simulink model "IEEE14_case"  (R2024b)
settings: Solver=FixedStepAuto  StartTime=0  StopTime=2  FixedStep=1e-7  RelTol=1e-3
values from neighbouring files (symbols this model uses):
  GFL_15_Bva = 0.009    [IEEE14_parameters.m]
  GFL_15_C_bus_pu = 7.179419    [IEEE14_parameters.m]
  GFL_15_f0 = 60    [IEEE14_parameters.m]
  GFL_15_I_id = 691.26967    [IEEE14_parameters.m]
  GFL_15_I_iq = 691.26967    [IEEE14_parameters.m]
  GFL_15_I_od = 45.2207    [IEEE14_parameters.m]
  GFL_15_I_oq = 45.2207    [IEEE14_parameters.m]
  GFL_15_I_pll = 0.78    [IEEE14_parameters.m]
  GFL_15_Kdi = 0.09    [IEEE14_parameters.m]
  GFL_15_Kdo = 0.9    [IEEE14_parameters.m]
  GFL_15_Kqi = 0.09    [IEEE14_parameters.m]
  GFL_15_Kqo = 0.9    [IEEE14_parameters.m]
  GFL_15_Lg_pu = 0.631447    [IEEE14_parameters.m]
  GFL_15_mode = 1    [IEEE14_parameters.m]
  GFL_15_P_id = 3.7166    [IEEE14_parameters.m]
  GFL_15_P_iq = 3.7166    [IEEE14_parameters.m]
  GFL_15_P_od = 0.4798    [IEEE14_parameters.m]
  GFL_15_P_oq = 0.4798    [IEEE14_parameters.m]
  GFL_15_P_pll = 290.42    [IEEE14_parameters.m]
  GFL_15_Qe_ref = 0.2    [IEEE14_parameters.m]
  GFL_15_Rg_pu = 0.024016    [IEEE14_parameters.m]
  GFL_15_Sbase = 1.000000e+4    (= 10000)    [IEEE14_parameters.m]
  GFL_15_Tdi = 0.01    [IEEE14_parameters.m]
  GFL_15_Tdo = 0.2    [IEEE14_parameters.m]
  GFL_15_Tqi = 0.01    [IEEE14_parameters.m]
  GFL_15_Tqo = 0.2    [IEEE14_parameters.m]
  GFL_15_Vbase = 380    [IEEE14_parameters.m]
  GFL_15_Vdc_ref = 1.011475    [IEEE14_parameters.m]
  GFL_15_Vdcbase = 700    [IEEE14_parameters.m]
  GFL_15_vq_ref = 0    [IEEE14_parameters.m]
  GFL_16_Bva = 0.002    [IEEE14_parameters.m]
  GFL_16_C_bus_pu = 7.179419    [IEEE14_parameters.m]
  GFL_16_f0 = 60    [IEEE14_parameters.m]
  GFL_16_I_id = 691.26967    [IEEE14_parameters.m]
  GFL_16_I_iq = 691.26967    [IEEE14_parameters.m]
  GFL_16_I_od = 45.2207    [IEEE14_parameters.m]
  GFL_16_I_oq = 45.2207    [IEEE14_parameters.m]
  GFL_16_I_pll = 0.78    [IEEE14_parameters.m]
  GFL_16_Kdi = 0.05    [IEEE14_parameters.m]
  GFL_16_Kdo = 0.5    [IEEE14_parameters.m]
  GFL_16_Kqi = 0.05    [IEEE14_parameters.m]
  GFL_16_Kqo = 0.5    [IEEE14_parameters.m]
  GFL_16_Lg_pu = 0.631447    [IEEE14_parameters.m]
  GFL_16_mode = 1    [IEEE14_parameters.m]
  GFL_16_P_id = 3.7166    [IEEE14_parameters.m]
  GFL_16_P_iq = 3.7166    [IEEE14_parameters.m]
  GFL_16_P_od = 0.4798    [IEEE14_parameters.m]
  GFL_16_P_oq = 0.4798    [IEEE14_parameters.m]
  GFL_16_P_pll = 290.42    [IEEE14_parameters.m]
  GFL_16_Qe_ref = 0.2    [IEEE14_parameters.m]
  GFL_16_Rg_pu = 0.024016    [IEEE14_parameters.m]
  GFL_16_Sbase = 1.000000e+4    (= 10000)    [IEEE14_parameters.m]
  GFL_16_Tdi = 0.01    [IEEE14_parameters.m]
  GFL_16_Tdo = 0.2    [IEEE14_parameters.m]
  GFL_16_Tqi = 0.01    [IEEE14_parameters.m]
  GFL_16_Tqo = 0.2    [IEEE14_parameters.m]
  GFL_16_Vbase = 380    [IEEE14_parameters.m]
  GFL_16_Vdc_ref = 1.01144    [IEEE14_parameters.m]
  GFL_16_Vdcbase = 700    [IEEE14_parameters.m]
  GFL_16_vq_ref = 0    [IEEE14_parameters.m]
  GFL_17_Bva = 0.002    [IEEE14_parameters.m]
  GFL_17_C_bus_pu = 7.179419    [IEEE14_parameters.m]
  GFL_17_f0 = 60    [IEEE14_parameters.m]
  GFL_17_I_id = 691.26967    [IEEE14_parameters.m]
  GFL_17_I_iq = 691.26967    [IEEE14_parameters.m]
  GFL_17_I_od = 45.2207    [IEEE14_parameters.m]
  GFL_17_I_oq = 45.2207    [IEEE14_parameters.m]
  GFL_17_I_pll = 0.78    [IEEE14_parameters.m]
  GFL_17_Kdi = 0.05    [IEEE14_parameters.m]
  GFL_17_Kdo = 0.5    [IEEE14_parameters.m]
  GFL_17_Kqi = 0.05    [IEEE14_parameters.m]
  GFL_17_Kqo = 0.5    [IEEE14_parameters.m]
  GFL_17_Lg_pu = 0.631447    [IEEE14_parameters.m]
  GFL_17_mode = 1    [IEEE14_parameters.m]
  GFL_17_P_id = 3.7166    [IEEE14_parameters.m]
  GFL_17_P_iq = 3.7166    [IEEE14_parameters.m]
  GFL_17_P_od = 0.4798    [IEEE14_parameters.m]
  GFL_17_P_oq = 0.4798    [IEEE14_parameters.m]
  GFL_17_P_pll = 290.42    [IEEE14_parameters.m]
  GFL_17_Qe_ref = 0.2    [IEEE14_parameters.m]
  GFL_17_Rg_pu = 0.024016    [IEEE14_parameters.m]
  GFL_17_Sbase = 1.000000e+4    (= 10000)    [IEEE14_parameters.m]
  GFL_17_Tdi = 0.01    [IEEE14_parameters.m]
  GFL_17_Tdo = 0.2    [IEEE14_parameters.m]
  GFL_17_Tqi = 0.01    [IEEE14_parameters.m]
  GFL_17_Tqo = 0.2    [IEEE14_parameters.m]
  GFL_17_Vbase = 380    [IEEE14_parameters.m]
  GFL_17_Vdc_ref = 1.011632    [IEEE14_parameters.m]
  GFL_17_Vdcbase = 700    [IEEE14_parameters.m]
  GFL_17_vq_ref = 0    [IEEE14_parameters.m]
  GFL_18_Bva = 0.002    [IEEE14_parameters.m]
  GFL_18_C_bus_pu = 7.179419    [IEEE14_parameters.m]
  GFL_18_f0 = 60    [IEEE14_parameters.m]
  GFL_18_I_id = 691.26967    [IEEE14_parameters.m]
  GFL_18_I_iq = 691.26967    [IEEE14_parameters.m]
  GFL_18_I_od = 45.2207    [IEEE14_parameters.m]
  GFL_18_I_oq = 45.2207    [IEEE14_parameters.m]
  GFL_18_I_pll = 0.78    [IEEE14_parameters.m]
  GFL_18_Kdi = 0.05    [IEEE14_parameters.m]
  GFL_18_Kdo = 0.5    [IEEE14_parameters.m]
  GFL_18_Kqi = 0.05    [IEEE14_parameters.m]
  GFL_18_Kqo = 0.5    [IEEE14_parameters.m]
  GFL_18_Lg_pu = 0.631447    [IEEE14_parameters.m]
  GFL_18_mode = 1    [IEEE14_parameters.m]
  GFL_18_P_id = 3.7166    [IEEE14_parameters.m]
  GFL_18_P_iq = 3.7166    [IEEE14_parameters.m]
  GFL_18_P_od = 0.4798    [IEEE14_parameters.m]
  GFL_18_P_oq = 0.4798    [IEEE14_parameters.m]
  GFL_18_P_pll = 290.42    [IEEE14_parameters.m]
  GFL_18_Qe_ref = 0.2    [IEEE14_parameters.m]
  GFL_18_Rg_pu = 0.024016    [IEEE14_parameters.m]
  GFL_18_Sbase = 1.000000e+4    (= 10000)    [IEEE14_parameters.m]
  GFL_18_Tdi = 0.01    [IEEE14_parameters.m]
  GFL_18_Tdo = 0.2    [IEEE14_parameters.m]
  GFL_18_Tqi = 0.01    [IEEE14_parameters.m]
  GFL_18_Tqo = 0.2    [IEEE14_parameters.m]
  GFL_18_Vbase = 380    [IEEE14_parameters.m]
  GFL_18_Vdc_ref = 1.011572    [IEEE14_parameters.m]
  GFL_18_Vdcbase = 700    [IEEE14_parameters.m]
  GFL_18_vq_ref = 0    [IEEE14_parameters.m]
  ... (+180 more)
(part 4 of 25)

== system IEEE14_case/SG_D_1 ==
  v_d_SG_D_1 : Inport
  v_q_SG_D_1 : Inport  Port=2
  E_fd_SG_D_1 : Integrator  InitialCondition=3.4212573415419114
  Px_1_SG_D_1 : Integrator  InitialCondition=0.0
  Px_2_SG_D_1 : Integrator  InitialCondition=0.0
  Px_3_SG_D_1 : Integrator  InitialCondition=-3.1830279294144415e-26
  R_f_SG_D_1 : Integrator  InitialCondition=23.098374565895817
  T_e_SG_D_1_block : Subsystem
  T_m_SG_D_1 : Integrator  InitialCondition=1.9014466706454893
  V_f_SG_D_1 : Integrator  InitialCondition=34.212573415419115
  d_E_fd_SG_D_1_block : Subsystem
  d_Px_1_SG_D_1_block : Subsystem
  d_Px_2_SG_D_1_block : Subsystem
  d_Px_3_SG_D_1_block : Subsystem
  d_R_f_SG_D_1_block : Subsystem
  d_T_m_SG_D_1_block : Subsystem
  d_V_f_SG_D_1_block : Subsystem
  d_psi_1d_SG_D_1_block : Subsystem
  d_psi_d_SG_D_1_block : Subsystem
  d_psi_fd_SG_D_1_block : Subsystem
  d_psi_gq_SG_D_1_block : Subsystem
  d_psi_kq_SG_D_1_block : Subsystem
  d_psi_q_SG_D_1_block : Subsystem
  d_theta_SG_D_1_block : Subsystem
  d_w_SG_D_1_block : Subsystem
  i_d_SG_D_1_block : Subsystem
  i_q_SG_D_1_block : Subsystem
  psi_1d_SG_D_1 : Integrator  InitialCondition=0.4032623891736521
  psi_d_SG_D_1 : Integrator  InitialCondition=0.32169495802856396
  psi_fd_SG_D_1 : Integrator  InitialCondition=0.8143622421448962
  psi_gq_SG_D_1 : Integrator  InitialCondition=0.6228002528652177
  psi_kq_SG_D_1 : Integrator  InitialCondition=-0.9731253951019027
  psi_q_SG_D_1 : Integrator  InitialCondition=-1.0120504109059787
  theta_SG_D_1 : Integrator  InitialCondition=1.263285946581872
  theta_SG_D_1_out_block : Subsystem
  w_SG_D_1 : Integrator  InitialCondition=376.99111843077515
  w_SG_D_1_out_block : Subsystem
  i_d_SG_D_1 : Outport
  i_q_SG_D_1 : Outport  Port=2
  T_e_SG_D_1 : Outport  Port=3
  w_SG_D_1_out : Outport  Port=4
  theta_SG_D_1_out : Outport  Port=5
  wires:
  d_theta_SG_D_1_block/1(Blockout_d_theta_SG_D_1_10b81) -> theta_SG_D_1/1
  V_f_SG_D_1/1 -> d_V_f_SG_D_1_block/14(State_V_f_SG_D_1_9a6da), d_E_fd_SG_D_1_block/2(State_V_f_SG_D_1_aa35b)
  psi_kq_SG_D_1/1 -> d_psi_q_SG_D_1_block/2(State_psi_kq_SG_D_1_494df), d_psi_gq_SG_D_1_block/3(State_psi_kq_SG_D_1_80cf5), d_psi_kq_SG_D_1_block/4(State_psi_kq_SG_D_1_7d6ac), d_psi_gq_SG_D_1_block/5(State_psi_kq_SG_D_1_884a1), d_V_f_SG_D_1_block/10(State_psi_kq_SG_D_1_02ae0), d_psi_gq_SG_D_1_block/8(State_psi_kq_SG_D_1_12411), i_d_SG_D_1_block/2(State_psi_kq_SG_D_1_0b4c3), d_psi_kq_SG_D_1_block/2(State_psi_kq_SG_D_1_b5070), T_e_SG_D_1_block/3(State_psi_kq_SG_D_1_246e1), i_q_SG_D_1_block/2(State_psi_kq_SG_D_1_fbc68), d_w_SG_D_1_block/5(State_psi_kq_SG_D_1_9c615)
  w_SG_D_1_out_block/1(Blockout_w_SG_D_1_out_d4c3b) -> w_SG_D_1_out/1
  d_Px_1_SG_D_1_block/1(Blockout_d_Px_1_SG_D_1_a4a61) -> Px_1_SG_D_1/1
  w_SG_D_1/1 -> d_V_f_SG_D_1_block/8(State_w_SG_D_1_7c0e0), d_psi_q_SG_D_1_block/9(State_w_SG_D_1_856b5), d_psi_d_SG_D_1_block/9(State_w_SG_D_1_7866a), d_V_f_SG_D_1_block/13(State_w_SG_D_1_d278a), d_T_m_SG_D_1_block/1(State_w_SG_D_1_4fd49), d_theta_SG_D_1_block/1(State_w_SG_D_1_d1dcd), d_Px_1_SG_D_1_block/2(State_w_SG_D_1_183d0), d_Px_2_SG_D_1_block/4(State_w_SG_D_1_83c31), d_w_SG_D_1_block/1(State_w_SG_D_1_bf0fb), d_Px_3_SG_D_1_block/6(State_w_SG_D_1_d6c43), w_SG_D_1_out_block/1(State_w_SG_D_1_b42d2)
  d_T_m_SG_D_1_block/1(Blockout_d_T_m_SG_D_1_8a3f6) -> T_m_SG_D_1/1
  d_Px_2_SG_D_1_block/1(Blockout_d_Px_2_SG_D_1_c2665) -> Px_2_SG_D_1/1
  d_Px_3_SG_D_1_block/1(Blockout_d_Px_3_SG_D_1_27eea) -> Px_3_SG_D_1/1
  psi_q_SG_D_1/1 -> d_psi_d_SG_D_1_block/8(State_psi_q_SG_D_1_339cd), d_psi_q_SG_D_1_block/3(State_psi_q_SG_D_1_68044), d_psi_gq_SG_D_1_block/6(State_psi_q_SG_D_1_99c8d), d_w_SG_D_1_block/7(State_psi_q_SG_D_1_36eb9), d_V_f_SG_D_1_block/11(State_psi_q_SG_D_1_7b289), i_d_SG_D_1_block/3(State_psi_q_SG_D_1_e8ece), d_w_SG_D_1_block/6(State_psi_q_SG_D_1_06dea), d_psi_gq_SG_D_1_block/9(State_psi_q_SG_D_1_31f88), i_q_SG_D_1_block/3(State_psi_q_SG_D_1_42b5e), d_V_f_SG_D_1_block/7(State_psi_q_SG_D_1_b21ce), d_psi_kq_SG_D_1_block/5(State_psi_q_SG_D_1_c6187), T_e_SG_D_1_block/4(State_psi_q_SG_D_1_fd30f), T_e_SG_D_1_block/5(State_psi_q_SG_D_1_04e42)
  psi_fd_SG_D_1/1 -> d_psi_fd_SG_D_1_block/2(State_psi_fd_SG_D_1_8f7d3), d_psi_fd_SG_D_1_block/10(State_psi_fd_SG_D_1_86724), d_psi_fd_SG_D_1_block/4(State_psi_fd_SG_D_1_d976b), d_psi_fd_SG_D_1_block/7(State_psi_fd_SG_D_1_c7a2f), d_psi_d_SG_D_1_block/3(State_psi_fd_SG_D_1_aad83), d_psi_1d_SG_D_1_block/5(State_psi_fd_SG_D_1_15435), d_w_SG_D_1_block/10(State_psi_fd_SG_D_1_a5e83), i_d_SG_D_1_block/7(State_psi_fd_SG_D_1_51096), i_q_SG_D_1_block/7(State_psi_fd_SG_D_1_ad572), d_V_f_SG_D_1_block/6(State_psi_fd_SG_D_1_fca9a), T_e_SG_D_1_block/8(State_psi_fd_SG_D_1_a5ec6), d_psi_1d_SG_D_1_block/2(State_psi_fd_SG_D_1_00af5)
  psi_gq_SG_D_1/1 -> d_psi_q_SG_D_1_block/1(State_psi_gq_SG_D_1_af930), d_psi_gq_SG_D_1_block/1(State_psi_gq_SG_D_1_6811c), d_psi_gq_SG_D_1_block/2(State_psi_gq_SG_D_1_53a5f), d_psi_gq_SG_D_1_block/7(State_psi_gq_SG_D_1_8041e), d_w_SG_D_1_block/4(State_psi_gq_SG_D_1_d212a), d_psi_kq_SG_D_1_block/1(State_psi_gq_SG_D_1_dba3b), i_d_SG_D_1_block/1(State_psi_gq_SG_D_1_8ae81), d_V_f_SG_D_1_block/9(State_psi_gq_SG_D_1_33342), d_psi_gq_SG_D_1_block/4(State_psi_gq_SG_D_1_5ed70), T_e_SG_D_1_block/2(State_psi_gq_SG_D_1_b91dd), i_q_SG_D_1_block/1(State_psi_gq_SG_D_1_70f72), d_psi_kq_SG_D_1_block/3(State_psi_gq_SG_D_1_cd69f)
  v_d_SG_D_1/1 -> d_psi_d_SG_D_1_block/4(Input_v_d_SG_D_1_751e0), d_psi_q_SG_D_1_block/4(Input_v_d_SG_D_1_3462f)
  T_m_SG_D_1/1 -> d_T_m_SG_D_1_block/2(State_T_m_SG_D_1_4e3cf), d_w_SG_D_1_block/2(State_T_m_SG_D_1_e0642)
  v_q_SG_D_1/1 -> d_psi_d_SG_D_1_block/6(Input_v_q_SG_D_1_569c6), d_psi_q_SG_D_1_block/6(Input_v_q_SG_D_1_86d27)
  Px_1_SG_D_1/1 -> d_Px_1_SG_D_1_block/1(State_Px_1_SG_D_1_41b99), d_Px_2_SG_D_1_block/3(State_Px_1_SG_D_1_ca7d0), d_Px_3_SG_D_1_block/4(State_Px_1_SG_D_1_d599f), d_Px_3_SG_D_1_block/5(State_Px_1_SG_D_1_5257c), d_Px_2_SG_D_1_block/2(State_Px_1_SG_D_1_02194)
  theta_SG_D_1/1 -> d_psi_d_SG_D_1_block/5(State_theta_SG_D_1_5b2d6), d_psi_q_SG_D_1_block/7(State_theta_SG_D_1_4261b), i_d_SG_D_1_block/4(State_theta_SG_D_1_02ca1), d_psi_d_SG_D_1_block/7(State_theta_SG_D_1_7d7a3), i_q_SG_D_1_block/4(State_theta_SG_D_1_4335e), d_psi_q_SG_D_1_block/5(State_theta_SG_D_1_16401), theta_SG_D_1_out_block/1(State_theta_SG_D_1_c8a88), i_q_SG_D_1_block/8(State_theta_SG_D_1_fd587), i_d_SG_D_1_block/8(State_theta_SG_D_1_8959d)
  Px_2_SG_D_1/1 -> d_Px_2_SG_D_1_block/1(State_Px_2_SG_D_1_52166), d_Px_3_SG_D_1_block/2(State_Px_2_SG_D_1_173b9), d_Px_3_SG_D_1_block/3(State_Px_2_SG_D_1_5b4c4)
  psi_d_SG_D_1/1 -> d_psi_fd_SG_D_1_block/9(State_psi_d_SG_D_1_5418d), d_psi_d_SG_D_1_block/2(State_psi_d_SG_D_1_b0cbd), d_psi_q_SG_D_1_block/8(State_psi_d_SG_D_1_ad817), d_w_SG_D_1_block/9(State_psi_d_SG_D_1_eab0d), d_w_SG_D_1_block/3(State_psi_d_SG_D_1_3bbbe), d_V_f_SG_D_1_block/5(State_psi_d_SG_D_1_3c550), d_psi_1d_SG_D_1_block/4(State_psi_d_SG_D_1_719b4), i_d_SG_D_1_block/6(State_psi_d_SG_D_1_e218a), i_q_SG_D_1_block/6(State_psi_d_SG_D_1_986bb), T_e_SG_D_1_block/1(State_psi_d_SG_D_1_5a569), d_V_f_SG_D_1_block/12(State_psi_d_SG_D_1_3754c), d_psi_fd_SG_D_1_block/6(State_psi_d_SG_D_1_eef22), T_e_SG_D_1_block/7(State_psi_d_SG_D_1_dfbb8)
  d_E_fd_SG_D_1_block/1(Blockout_d_E_fd_SG_D_1_7b54f) -> E_fd_SG_D_1/1
  psi_1d_SG_D_1/1 -> d_psi_fd_SG_D_1_block/3(State_psi_1d_SG_D_1_1898e), d_psi_fd_SG_D_1_block/8(State_psi_1d_SG_D_1_2c9f9), d_psi_d_SG_D_1_block/1(State_psi_1d_SG_D_1_69d00), d_psi_1d_SG_D_1_block/3(State_psi_1d_SG_D_1_c5f75), d_V_f_SG_D_1_block/4(State_psi_1d_SG_D_1_6838f), i_d_SG_D_1_block/5(State_psi_1d_SG_D_1_6fa9d), d_w_SG_D_1_block/8(State_psi_1d_SG_D_1_bb43d), i_q_SG_D_1_block/5(State_psi_1d_SG_D_1_63ddd), d_psi_1d_SG_D_1_block/1(State_psi_1d_SG_D_1_959f0), T_e_SG_D_1_block/6(State_psi_1d_SG_D_1_ba9b8), d_psi_fd_SG_D_1_block/5(State_psi_1d_SG_D_1_f6ad7)
  d_V_f_SG_D_1_block/1(Blockout_d_V_f_SG_D_1_61597) -> V_f_SG_D_1/1
  d_psi_q_SG_D_1_block/1(Blockout_d_psi_q_SG_D_1_f8953) -> psi_q_SG_D_1/1
  d_psi_gq_SG_D_1_block/1(Blockout_d_psi_gq_SG_D_1_56070) -> psi_gq_SG_D_1/1
  theta_SG_D_1_out_block/1(Blockout_theta_SG_D_1_out_3d7c0) -> theta_SG_D_1_out/1
  d_R_f_SG_D_1_block/1(Blockout_d_R_f_SG_D_1_dc367) -> R_f_SG_D_1/1
  d_w_SG_D_1_block/1(Blockout_d_w_SG_D_1_3fcfa) -> w_SG_D_1/1
  T_e_SG_D_1_block/1(Blockout_T_e_SG_D_1_52337) -> T_e_SG_D_1/1
  d_psi_d_SG_D_1_block/1(Blockout_d_psi_d_SG_D_1_2cdbf) -> psi_d_SG_D_1/1
  d_psi_kq_SG_D_1_block/1(Blockout_d_psi_kq_SG_D_1_d51b4) -> psi_kq_SG_D_1/1
  i_q_SG_D_1_block/1(Blockout_i_q_SG_D_1_04b1b) -> i_q_SG_D_1/1
  i_d_SG_D_1_block/1(Blockout_i_d_SG_D_1_f5e95) -> i_d_SG_D_1/1
  d_psi_1d_SG_D_1_block/1(Blockout_d_psi_1d_SG_D_1_ce82a) -> psi_1d_SG_D_1/1
  Px_3_SG_D_1/1 -> d_V_f_SG_D_1_block/3(State_Px_3_SG_D_1_35ab0), d_Px_3_SG_D_1_block/1(State_Px_3_SG_D_1_65e83)
  R_f_SG_D_1/1 -> d_V_f_SG_D_1_block/2(State_R_f_SG_D_1_39127), d_R_f_SG_D_1_block/2(State_R_f_SG_D_1_c9358)
  E_fd_SG_D_1/1 -> d_V_f_SG_D_1_block/1(State_E_fd_SG_D_1_b54d1), d_E_fd_SG_D_1_block/1(State_E_fd_SG_D_1_314b1), d_R_f_SG_D_1_block/1(State_E_fd_SG_D_1_43088), d_psi_fd_SG_D_1_block/1(State_E_fd_SG_D_1_05819)
  d_psi_fd_SG_D_1_block/1(Blockout_d_psi_fd_SG_D_1_936e9) -> psi_fd_SG_D_1/1

== system IEEE14_case/SG_D_2 ==
  v_d_SG_D_2 : Inport
  v_q_SG_D_2 : Inport  Port=2
  E_fd_SG_D_2 : Integrator  InitialCondition=1.1780887532081583
  Px_1_SG_D_2 : Integrator  InitialCondition=0.0
  Px_2_SG_D_2 : Integrator  InitialCondition=0.0
  Px_3_SG_D_2 : Integrator  InitialCondition=-1.1116920340485189e-30
  R_f_SG_D_2 : Integrator  InitialCondition=7.953782068088223
  T_e_SG_D_2_block : Subsystem
  T_m_SG_D_2 : Integrator  InitialCondition=0.40016203494093494
  V_f_SG_D_2 : Integrator  InitialCondition=11.780887532081582
  d_E_fd_SG_D_2_block : Subsystem
  d_Px_1_SG_D_2_block : Subsystem
  d_Px_2_SG_D_2_block : Subsystem
  d_Px_3_SG_D_2_block : Subsystem
  d_R_f_SG_D_2_block : Subsystem
  d_T_m_SG_D_2_block : Subsystem
  d_V_f_SG_D_2_block : Subsystem
  d_psi_1d_SG_D_2_block : Subsystem
  d_psi_d_SG_D_2_block : Subsystem
  d_psi_fd_SG_D_2_block : Subsystem
  d_psi_gq_SG_D_2_block : Subsystem
  d_psi_kq_SG_D_2_block : Subsystem
  d_psi_q_SG_D_2_block : Subsystem
  d_theta_SG_D_2_block : Subsystem
  d_w_SG_D_2_block : Subsystem
  i_d_SG_D_2_block : Subsystem
  i_q_SG_D_2_block : Subsystem
  psi_1d_SG_D_2 : Integrator  InitialCondition=0.9389092187130986
  psi_d_SG_D_2 : Integrator  InitialCondition=0.9324449069699886
  psi_fd_SG_D_2 : Integrator  InitialCondition=0.9714893498983717
  psi_gq_SG_D_2 : Integrator  InitialCondition=0.290890212850531
  psi_kq_SG_D_2 : Integrator  InitialCondition=-0.45451595757895474
  psi_q_SG_D_2 : Integrator  InitialCondition=-0.47269659588211294
  theta_SG_D_2 : Integrator  InitialCondition=0.39900394090305374
  theta_SG_D_2_out_block : Subsystem
  w_SG_D_2 : Integrator  InitialCondition=376.99111843077515
  w_SG_D_2_out_block : Subsystem
  i_d_SG_D_2 : Outport
  i_q_SG_D_2 : Outport  Port=2
  T_e_SG_D_2 : Outport  Port=3
  w_SG_D_2_out : Outport  Port=4
  theta_SG_D_2_out : Outport  Port=5
  wires:
  T_e_SG_D_2_block/1(Blockout_T_e_SG_D_2_7a393) -> T_e_SG_D_2/1
  d_Px_2_SG_D_2_block/1(Blockout_d_Px_2_SG_D_2_dd680) -> Px_2_SG_D_2/1
  d_T_m_SG_D_2_block/1(Blockout_d_T_m_SG_D_2_a859c) -> T_m_SG_D_2/1
  w_SG_D_2/1 -> d_psi_d_SG_D_2_block/9(State_w_SG_D_2_3bf29), d_w_SG_D_2_block/1(State_w_SG_D_2_04eee), d_V_f_SG_D_2_block/8(State_w_SG_D_2_66c76), d_psi_q_SG_D_2_block/9(State_w_SG_D_2_ecb88), d_V_f_SG_D_2_block/13(State_w_SG_D_2_ea751), d_theta_SG_D_2_block/1(State_w_SG_D_2_44e1a), d_T_m_SG_D_2_block/1(State_w_SG_D_2_28412), d_Px_2_SG_D_2_block/4(State_w_SG_D_2_0c27f), d_Px_3_SG_D_2_block/6(State_w_SG_D_2_29f15), d_Px_1_SG_D_2_block/2(State_w_SG_D_2_57c67), w_SG_D_2_out_block/1(State_w_SG_D_2_35bfa)
  psi_q_SG_D_2/1 -> d_psi_d_SG_D_2_block/8(State_psi_q_SG_D_2_54a7c), d_psi_q_SG_D_2_block/3(State_psi_q_SG_D_2_b05c7), d_psi_gq_SG_D_2_block/6(State_psi_q_SG_D_2_c887c), d_psi_gq_SG_D_2_block/9(State_psi_q_SG_D_2_400a1), d_psi_kq_SG_D_2_block/5(State_psi_q_SG_D_2_cfb7c), d_w_SG_D_2_block/7(State_psi_q_SG_D_2_8635e), d_V_f_SG_D_2_block/7(State_psi_q_SG_D_2_698d7), i_d_SG_D_2_block/3(State_psi_q_SG_D_2_b30b5), T_e_SG_D_2_block/4(State_psi_q_SG_D_2_7be04), i_q_SG_D_2_block/3(State_psi_q_SG_D_2_38e4d), d_w_SG_D_2_block/6(State_psi_q_SG_D_2_03373), T_e_SG_D_2_block/5(State_psi_q_SG_D_2_caf2c), d_V_f_SG_D_2_block/11(State_psi_q_SG_D_2_de371)
  w_SG_D_2_out_block/1(Blockout_w_SG_D_2_out_7dd39) -> w_SG_D_2_out/1
  T_m_SG_D_2/1 -> d_T_m_SG_D_2_block/2(State_T_m_SG_D_2_839d4), d_w_SG_D_2_block/2(State_T_m_SG_D_2_0748f)
  d_theta_SG_D_2_block/1(Blockout_d_theta_SG_D_2_e87fa) -> theta_SG_D_2/1
  d_Px_1_SG_D_2_block/1(Blockout_d_Px_1_SG_D_2_466a7) -> Px_1_SG_D_2/1
  d_Px_3_SG_D_2_block/1(Blockout_d_Px_3_SG_D_2_c9fb9) -> Px_3_SG_D_2/1
  Px_2_SG_D_2/1 -> d_Px_2_SG_D_2_block/1(State_Px_2_SG_D_2_863da), d_Px_3_SG_D_2_block/2(State_Px_2_SG_D_2_b3dc6), d_Px_3_SG_D_2_block/3(State_Px_2_SG_D_2_577d6)
  theta_SG_D_2/1 -> d_psi_d_SG_D_2_block/5(State_theta_SG_D_2_fba08), d_psi_q_SG_D_2_block/5(State_theta_SG_D_2_ba654), i_d_SG_D_2_block/4(State_theta_SG_D_2_acd34), d_psi_q_SG_D_2_block/7(State_theta_SG_D_2_5db71), i_d_SG_D_2_block/8(State_theta_SG_D_2_fc4e1), i_q_SG_D_2_block/4(State_theta_SG_D_2_4758d), i_q_SG_D_2_block/8(State_theta_SG_D_2_47d8a), theta_SG_D_2_out_block/1(State_theta_SG_D_2_36941), d_psi_d_SG_D_2_block/7(State_theta_SG_D_2_1738b)
  i_d_SG_D_2_block/1(Blockout_i_d_SG_D_2_ab50a) -> i_d_SG_D_2/1
  psi_d_SG_D_2/1 -> d_psi_fd_SG_D_2_block/6(State_psi_d_SG_D_2_1798b), d_psi_fd_SG_D_2_block/9(State_psi_d_SG_D_2_c30ab), d_psi_q_SG_D_2_block/8(State_psi_d_SG_D_2_4f2c3), d_psi_1d_SG_D_2_block/4(State_psi_d_SG_D_2_f297a), d_w_SG_D_2_block/3(State_psi_d_SG_D_2_6ae82), d_w_SG_D_2_block/9(State_psi_d_SG_D_2_d3800), d_psi_d_SG_D_2_block/2(State_psi_d_SG_D_2_46d33), d_V_f_SG_D_2_block/12(State_psi_d_SG_D_2_35745), i_d_SG_D_2_block/6(State_psi_d_SG_D_2_21b88), i_q_SG_D_2_block/6(State_psi_d_SG_D_2_afab4), d_V_f_SG_D_2_block/5(State_psi_d_SG_D_2_fc0d8), T_e_SG_D_2_block/1(State_psi_d_SG_D_2_5317f), T_e_SG_D_2_block/7(State_psi_d_SG_D_2_ed23a)
  psi_1d_SG_D_2/1 -> d_psi_fd_SG_D_2_block/5(State_psi_1d_SG_D_2_c8d78), d_psi_fd_SG_D_2_block/8(State_psi_1d_SG_D_2_e893c), d_psi_fd_SG_D_2_block/3(State_psi_1d_SG_D_2_84bab), d_psi_1d_SG_D_2_block/1(State_psi_1d_SG_D_2_5768c), d_V_f_SG_D_2_block/4(State_psi_1d_SG_D_2_cce5d), d_w_SG_D_2_block/8(State_psi_1d_SG_D_2_3458c), i_d_SG_D_2_block/5(State_psi_1d_SG_D_2_9c394), i_q_SG_D_2_block/5(State_psi_1d_SG_D_2_da86a), d_psi_d_SG_D_2_block/1(State_psi_1d_SG_D_2_d5455), T_e_SG_D_2_block/6(State_psi_1d_SG_D_2_2fd39), d_psi_1d_SG_D_2_block/3(State_psi_1d_SG_D_2_34f10)
  psi_kq_SG_D_2/1 -> d_psi_q_SG_D_2_block/2(State_psi_kq_SG_D_2_3a32d), d_psi_gq_SG_D_2_block/3(State_psi_kq_SG_D_2_229b6), d_psi_gq_SG_D_2_block/5(State_psi_kq_SG_D_2_a4801), d_psi_kq_SG_D_2_block/2(State_psi_kq_SG_D_2_f7bb1), d_V_f_SG_D_2_block/10(State_psi_kq_SG_D_2_9c81b), d_w_SG_D_2_block/5(State_psi_kq_SG_D_2_19d78), i_d_SG_D_2_block/2(State_psi_kq_SG_D_2_eeb5f), d_psi_kq_SG_D_2_block/4(State_psi_kq_SG_D_2_18fe7), i_q_SG_D_2_block/2(State_psi_kq_SG_D_2_485e8), d_psi_gq_SG_D_2_block/8(State_psi_kq_SG_D_2_c4824), T_e_SG_D_2_block/3(State_psi_kq_SG_D_2_8eee7)
  v_d_SG_D_2/1 -> d_psi_q_SG_D_2_block/4(Input_v_d_SG_D_2_1b10e), d_psi_d_SG_D_2_block/4(Input_v_d_SG_D_2_d6dc0)
  d_V_f_SG_D_2_block/1(Blockout_d_V_f_SG_D_2_c52b2) -> V_f_SG_D_2/1
  v_q_SG_D_2/1 -> d_psi_d_SG_D_2_block/6(Input_v_q_SG_D_2_00db2), d_psi_q_SG_D_2_block/6(Input_v_q_SG_D_2_876cf)
  Px_1_SG_D_2/1 -> d_Px_1_SG_D_2_block/1(State_Px_1_SG_D_2_416e3), d_Px_2_SG_D_2_block/2(State_Px_1_SG_D_2_cbeb2), d_Px_3_SG_D_2_block/4(State_Px_1_SG_D_2_b7377), d_Px_3_SG_D_2_block/5(State_Px_1_SG_D_2_616ef), d_Px_2_SG_D_2_block/3(State_Px_1_SG_D_2_01235)
  psi_fd_SG_D_2/1 -> d_psi_fd_SG_D_2_block/2(State_psi_fd_SG_D_2_2df35), d_psi_fd_SG_D_2_block/4(State_psi_fd_SG_D_2_f521e), d_psi_fd_SG_D_2_block/10(State_psi_fd_SG_D_2_fdcf2), d_psi_d_SG_D_2_block/3(State_psi_fd_SG_D_2_e734d), d_psi_fd_SG_D_2_block/7(State_psi_fd_SG_D_2_82c24), d_psi_1d_SG_D_2_block/5(State_psi_fd_SG_D_2_c105c), d_w_SG_D_2_block/10(State_psi_fd_SG_D_2_b728a), d_V_f_SG_D_2_block/6(State_psi_fd_SG_D_2_82b8b), i_d_SG_D_2_block/7(State_psi_fd_SG_D_2_34aa6), i_q_SG_D_2_block/7(State_psi_fd_SG_D_2_93752), d_psi_1d_SG_D_2_block/2(State_psi_fd_SG_D_2_4ee86), T_e_SG_D_2_block/8(State_psi_fd_SG_D_2_ca537)
  psi_gq_SG_D_2/1 -> d_psi_gq_SG_D_2_block/1(State_psi_gq_SG_D_2_f404a), d_psi_gq_SG_D_2_block/2(State_psi_gq_SG_D_2_79e41), d_psi_gq_SG_D_2_block/4(State_psi_gq_SG_D_2_41ece), d_psi_q_SG_D_2_block/1(State_psi_gq_SG_D_2_7a17f), d_psi_gq_SG_D_2_block/7(State_psi_gq_SG_D_2_c13c7), d_psi_kq_SG_D_2_block/3(State_psi_gq_SG_D_2_cbe5c), d_psi_kq_SG_D_2_block/1(State_psi_gq_SG_D_2_f92a1), d_V_f_SG_D_2_block/9(State_psi_gq_SG_D_2_505e8), i_d_SG_D_2_block/1(State_psi_gq_SG_D_2_24483), i_q_SG_D_2_block/1(State_psi_gq_SG_D_2_7930d), d_w_SG_D_2_block/4(State_psi_gq_SG_D_2_fb75f), T_e_SG_D_2_block/2(State_psi_gq_SG_D_2_6936d)
  d_R_f_SG_D_2_block/1(Blockout_d_R_f_SG_D_2_1f586) -> R_f_SG_D_2/1
  d_psi_1d_SG_D_2_block/1(Blockout_d_psi_1d_SG_D_2_81873) -> psi_1d_SG_D_2/1
  i_q_SG_D_2_block/1(Blockout_i_q_SG_D_2_d03bb) -> i_q_SG_D_2/1
  R_f_SG_D_2/1 -> d_V_f_SG_D_2_block/2(State_R_f_SG_D_2_b9cb8), d_R_f_SG_D_2_block/2(State_R_f_SG_D_2_a3c1e)
  theta_SG_D_2_out_block/1(Blockout_theta_SG_D_2_out_85337) -> theta_SG_D_2_out/1
  d_w_SG_D_2_block/1(Blockout_d_w_SG_D_2_78b05) -> w_SG_D_2/1
  d_psi_kq_SG_D_2_block/1(Blockout_d_psi_kq_SG_D_2_03e6e) -> psi_kq_SG_D_2/1
  d_psi_d_SG_D_2_block/1(Blockout_d_psi_d_SG_D_2_bb4d6) -> psi_d_SG_D_2/1
  d_psi_q_SG_D_2_block/1(Blockout_d_psi_q_SG_D_2_a5b60) -> psi_q_SG_D_2/1
  d_psi_gq_SG_D_2_block/1(Blockout_d_psi_gq_SG_D_2_f3eae) -> psi_gq_SG_D_2/1
  V_f_SG_D_2/1 -> d_V_f_SG_D_2_block/14(State_V_f_SG_D_2_63df0), d_E_fd_SG_D_2_block/2(State_V_f_SG_D_2_6e69e)
  Px_3_SG_D_2/1 -> d_V_f_SG_D_2_block/3(State_Px_3_SG_D_2_c6f53), d_Px_3_SG_D_2_block/1(State_Px_3_SG_D_2_18957)
  d_E_fd_SG_D_2_block/1(Blockout_d_E_fd_SG_D_2_3931e) -> E_fd_SG_D_2/1
  E_fd_SG_D_2/1 -> d_V_f_SG_D_2_block/1(State_E_fd_SG_D_2_5887d), d_R_f_SG_D_2_block/1(State_E_fd_SG_D_2_d9efc), d_E_fd_SG_D_2_block/1(State_E_fd_SG_D_2_0281f), d_psi_fd_SG_D_2_block/1(State_E_fd_SG_D_2_01a4d)
  d_psi_fd_SG_D_2_block/1(Blockout_d_psi_fd_SG_D_2_ab69d) -> psi_fd_SG_D_2/1

== system IEEE14_case/SG_D_3 ==
  v_d_SG_D_3 : Inport
  v_q_SG_D_3 : Inport  Port=2
  E_fd_SG_D_3 : Integrator  InitialCondition=1.097270100445358
  Px_1_SG_D_3 : Integrator  InitialCondition=0.0
  Px_2_SG_D_3 : Integrator  InitialCondition=0.0
  Px_3_SG_D_3 : Integrator  InitialCondition=-1.1312416114872206e-28
  R_f_SG_D_3 : Integrator  InitialCondition=7.408140706721088
  T_e_SG_D_3_block : Subsystem
  T_m_SG_D_3 : Integrator  InitialCondition=2.295378381999633e-06
  V_f_SG_D_3 : Integrator  InitialCondition=10.972701004453581
  d_E_fd_SG_D_3_block : Subsystem
  d_Px_1_SG_D_3_block : Subsystem
  d_Px_2_SG_D_3_block : Subsystem
  d_Px_3_SG_D_3_block : Subsystem
  d_R_f_SG_D_3_block : Subsystem
  d_T_m_SG_D_3_block : Subsystem
  d_V_f_SG_D_3_block : Subsystem
  d_psi_1d_SG_D_3_block : Subsystem
  d_psi_d_SG_D_3_block : Subsystem
  d_psi_fd_SG_D_3_block : Subsystem
  d_psi_gq_SG_D_3_block : Subsystem
  d_psi_kq_SG_D_3_block : Subsystem
  d_psi_q_SG_D_3_block : Subsystem
  d_theta_SG_D_3_block : Subsystem
  d_w_SG_D_3_block : Subsystem
  i_d_SG_D_3_block : Subsystem
  i_q_SG_D_3_block : Subsystem
  psi_1d_SG_D_3 : Integrator  InitialCondition=1.0122965827875312
  psi_d_SG_D_3 : Integrator  InitialCondition=1.0100000012292114
  psi_fd_SG_D_3 : Integrator  InitialCondition=1.0238713538414623
  psi_gq_SG_D_3 : Integrator  InitialCondition=1.7166577732193318e-06
  psi_kq_SG_D_3 : Integrator  InitialCondition=-2.6822777706538834e-06
  psi_q_SG_D_3 : Integrator  InitialCondition=-2.7895688814801745e-06
  theta_SG_D_3 : Integrator  InitialCondition=-0.1923744826171874
  theta_SG_D_3_out_block : Subsystem
  w_SG_D_3 : Integrator  InitialCondition=376.99111843077515
  w_SG_D_3_out_block : Subsystem
  i_d_SG_D_3 : Outport
  i_q_SG_D_3 : Outport  Port=2
  T_e_SG_D_3 : Outport  Port=3
  w_SG_D_3_out : Outport  Port=4
  theta_SG_D_3_out : Outport  Port=5
  wires:
  d_Px_1_SG_D_3_block/1(Blockout_d_Px_1_SG_D_3_2db33) -> Px_1_SG_D_3/1
  w_SG_D_3/1 -> d_psi_d_SG_D_3_block/9(State_w_SG_D_3_cf454), d_psi_q_SG_D_3_block/9(State_w_SG_D_3_3bc6e), d_w_SG_D_3_block/1(State_w_SG_D_3_2376b), d_V_f_SG_D_3_block/13(State_w_SG_D_3_51c21), d_V_f_SG_D_3_block/8(State_w_SG_D_3_75712), d_theta_SG_D_3_block/1(State_w_SG_D_3_b92e8), d_T_m_SG_D_3_block/1(State_w_SG_D_3_dca15), d_Px_2_SG_D_3_block/4(State_w_SG_D_3_c1cd3), d_Px_1_SG_D_3_block/2(State_w_SG_D_3_8df22), d_Px_3_SG_D_3_block/6(State_w_SG_D_3_40967), w_SG_D_3_out_block/1(State_w_SG_D_3_f6ed4)
  psi_fd_SG_D_3/1 -> d_psi_fd_SG_D_3_block/2(State_psi_fd_SG_D_3_1ca94), d_psi_fd_SG_D_3_block/7(State_psi_fd_SG_D_3_13cfd), d_psi_fd_SG_D_3_block/10(State_psi_fd_SG_D_3_01d8a), d_psi_d_SG_D_3_block/3(State_psi_fd_SG_D_3_dc857), d_V_f_SG_D_3_block/6(State_psi_fd_SG_D_3_9ff99), i_d_SG_D_3_block/7(State_psi_fd_SG_D_3_32316), d_w_SG_D_3_block/10(State_psi_fd_SG_D_3_2ef0f), i_q_SG_D_3_block/7(State_psi_fd_SG_D_3_bfdd7), d_psi_1d_SG_D_3_block/5(State_psi_fd_SG_D_3_e270b), T_e_SG_D_3_block/8(State_psi_fd_SG_D_3_2a972), d_psi_fd_SG_D_3_block/4(State_psi_fd_SG_D_3_1fedc), d_psi_1d_SG_D_3_block/2(State_psi_fd_SG_D_3_a754d)
  d_Px_3_SG_D_3_block/1(Blockout_d_Px_3_SG_D_3_533e8) -> Px_3_SG_D_3/1
  R_f_SG_D_3/1 -> d_R_f_SG_D_3_block/2(State_R_f_SG_D_3_eb135), d_V_f_SG_D_3_block/2(State_R_f_SG_D_3_bcbbe)
  w_SG_D_3_out_block/1(Blockout_w_SG_D_3_out_ef88e) -> w_SG_D_3_out/1
  d_Px_2_SG_D_3_block/1(Blockout_d_Px_2_SG_D_3_ebaee) -> Px_2_SG_D_3/1
  d_T_m_SG_D_3_block/1(Blockout_d_T_m_SG_D_3_ccb21) -> T_m_SG_D_3/1
  d_w_SG_D_3_block/1(Blockout_d_w_SG_D_3_aa189) -> w_SG_D_3/1
  Px_1_SG_D_3/1 -> d_Px_1_SG_D_3_block/1(State_Px_1_SG_D_3_31f88), d_Px_3_SG_D_3_block/4(State_Px_1_SG_D_3_ffa71), d_Px_3_SG_D_3_block/5(State_Px_1_SG_D_3_1185a), d_Px_2_SG_D_3_block/2(State_Px_1_SG_D_3_9548d), d_Px_2_SG_D_3_block/3(State_Px_1_SG_D_3_76f6d)
  d_theta_SG_D_3_block/1(Blockout_d_theta_SG_D_3_c1b15) -> theta_SG_D_3/1
  d_psi_kq_SG_D_3_block/1(Blockout_d_psi_kq_SG_D_3_bc348) -> psi_kq_SG_D_3/1
  psi_1d_SG_D_3/1 -> d_psi_fd_SG_D_3_block/3(State_psi_1d_SG_D_3_100d0), d_psi_fd_SG_D_3_block/5(State_psi_1d_SG_D_3_43bed), d_psi_fd_SG_D_3_block/8(State_psi_1d_SG_D_3_3ce6e), d_psi_d_SG_D_3_block/1(State_psi_1d_SG_D_3_784cd), d_psi_1d_SG_D_3_block/1(State_psi_1d_SG_D_3_7e8a3), d_w_SG_D_3_block/8(State_psi_1d_SG_D_3_c9bae), d_V_f_SG_D_3_block/4(State_psi_1d_SG_D_3_1255a), i_d_SG_D_3_block/5(State_psi_1d_SG_D_3_f1d32), d_psi_1d_SG_D_3_block/3(State_psi_1d_SG_D_3_1b7c5), i_q_SG_D_3_block/5(State_psi_1d_SG_D_3_20d6e), T_e_SG_D_3_block/6(State_psi_1d_SG_D_3_7e2e9)
  psi_kq_SG_D_3/1 -> d_psi_gq_SG_D_3_block/3(State_psi_kq_SG_D_3_dfb0b), d_psi_gq_SG_D_3_block/5(State_psi_kq_SG_D_3_5ef0d), d_psi_kq_SG_D_3_block/2(State_psi_kq_SG_D_3_66cec), d_psi_gq_SG_D_3_block/8(State_psi_kq_SG_D_3_da800), i_d_SG_D_3_block/2(State_psi_kq_SG_D_3_79fd4), i_q_SG_D_3_block/2(State_psi_kq_SG_D_3_3c737), d_w_SG_D_3_block/5(State_psi_kq_SG_D_3_d40a5), d_psi_kq_SG_D_3_block/4(State_psi_kq_SG_D_3_3bd28), d_psi_q_SG_D_3_block/2(State_psi_kq_SG_D_3_9869f), d_V_f_SG_D_3_block/10(State_psi_kq_SG_D_3_be735), T_e_SG_D_3_block/3(State_psi_kq_SG_D_3_a8962)
  Px_2_SG_D_3/1 -> d_Px_3_SG_D_3_block/3(State_Px_2_SG_D_3_bc145), d_Px_2_SG_D_3_block/1(State_Px_2_SG_D_3_c0631), d_Px_3_SG_D_3_block/2(State_Px_2_SG_D_3_c14d3)
  T_m_SG_D_3/1 -> d_T_m_SG_D_3_block/2(State_T_m_SG_D_3_13cc0), d_w_SG_D_3_block/2(State_T_m_SG_D_3_41b09)
  psi_gq_SG_D_3/1 -> d_psi_q_SG_D_3_block/1(State_psi_gq_SG_D_3_7cee6), d_psi_gq_SG_D_3_block/1(State_psi_gq_SG_D_3_61d89), d_psi_gq_SG_D_3_block/2(State_psi_gq_SG_D_3_d2fbb), d_psi_gq_SG_D_3_block/4(State_psi_gq_SG_D_3_45fb4), d_V_f_SG_D_3_block/9(State_psi_gq_SG_D_3_fc19e), d_psi_gq_SG_D_3_block/7(State_psi_gq_SG_D_3_a842f), i_d_SG_D_3_block/1(State_psi_gq_SG_D_3_ef59b), i_q_SG_D_3_block/1(State_psi_gq_SG_D_3_f7c17), d_w_SG_D_3_block/4(State_psi_gq_SG_D_3_2aa1e), d_psi_kq_SG_D_3_block/1(State_psi_gq_SG_D_3_5f103), T_e_SG_D_3_block/2(State_psi_gq_SG_D_3_9f172), d_psi_kq_SG_D_3_block/3(State_psi_gq_SG_D_3_d768f)
  v_d_SG_D_3/1 -> d_psi_q_SG_D_3_block/4(Input_v_d_SG_D_3_62f18), d_psi_d_SG_D_3_block/4(Input_v_d_SG_D_3_50bcc)
  v_q_SG_D_3/1 -> d_psi_d_SG_D_3_block/6(Input_v_q_SG_D_3_cd8a7), d_psi_q_SG_D_3_block/6(Input_v_q_SG_D_3_5442f)
  psi_q_SG_D_3/1 -> d_psi_d_SG_D_3_block/8(State_psi_q_SG_D_3_52034), d_psi_gq_SG_D_3_block/6(State_psi_q_SG_D_3_2ea70), d_psi_gq_SG_D_3_block/9(State_psi_q_SG_D_3_77fff), d_psi_q_SG_D_3_block/3(State_psi_q_SG_D_3_e7c3e), d_psi_kq_SG_D_3_block/5(State_psi_q_SG_D_3_41969), d_V_f_SG_D_3_block/7(State_psi_q_SG_D_3_41f04), d_V_f_SG_D_3_block/11(State_psi_q_SG_D_3_ccb6a), d_w_SG_D_3_block/7(State_psi_q_SG_D_3_f6aa0), i_d_SG_D_3_block/3(State_psi_q_SG_D_3_6a903), d_w_SG_D_3_block/6(State_psi_q_SG_D_3_648aa), i_q_SG_D_3_block/3(State_psi_q_SG_D_3_2676a), T_e_SG_D_3_block/4(State_psi_q_SG_D_3_e8f69), T_e_SG_D_3_block/5(State_psi_q_SG_D_3_454dd)
  theta_SG_D_3/1 -> d_psi_d_SG_D_3_block/5(State_theta_SG_D_3_e69f1), d_psi_q_SG_D_3_block/5(State_theta_SG_D_3_1d26c), i_d_SG_D_3_block/4(State_theta_SG_D_3_fed8f), i_d_SG_D_3_block/8(State_theta_SG_D_3_96b23), i_q_SG_D_3_block/4(State_theta_SG_D_3_9134c), d_psi_q_SG_D_3_block/7(State_theta_SG_D_3_b7f72), i_q_SG_D_3_block/8(State_theta_SG_D_3_28037), theta_SG_D_3_out_block/1(State_theta_SG_D_3_9fa07), d_psi_d_SG_D_3_block/7(State_theta_SG_D_3_09dff)
  psi_d_SG_D_3/1 -> d_psi_fd_SG_D_3_block/6(State_psi_d_SG_D_3_d3054), d_psi_fd_SG_D_3_block/9(State_psi_d_SG_D_3_4847b), d_psi_d_SG_D_3_block/2(State_psi_d_SG_D_3_c3430), d_psi_q_SG_D_3_block/8(State_psi_d_SG_D_3_6630b), d_psi_1d_SG_D_3_block/4(State_psi_d_SG_D_3_3e6ac), d_w_SG_D_3_block/3(State_psi_d_SG_D_3_bb520), d_V_f_SG_D_3_block/5(State_psi_d_SG_D_3_9a24c), d_V_f_SG_D_3_block/12(State_psi_d_SG_D_3_1ea12), i_q_SG_D_3_block/6(State_psi_d_SG_D_3_ac680), i_d_SG_D_3_block/6(State_psi_d_SG_D_3_cc5ad), T_e_SG_D_3_block/1(State_psi_d_SG_D_3_0fe66), d_w_SG_D_3_block/9(State_psi_d_SG_D_3_02a5f), T_e_SG_D_3_block/7(State_psi_d_SG_D_3_9c5b0)
  theta_SG_D_3_out_block/1(Blockout_theta_SG_D_3_out_2c966) -> theta_SG_D_3_out/1
  d_V_f_SG_D_3_block/1(Blockout_d_V_f_SG_D_3_1ea6f) -> V_f_SG_D_3/1
  d_psi_q_SG_D_3_block/1(Blockout_d_psi_q_SG_D_3_309b6) -> psi_q_SG_D_3/1
  d_R_f_SG_D_3_block/1(Blockout_d_R_f_SG_D_3_2588d) -> R_f_SG_D_3/1
  T_e_SG_D_3_block/1(Blockout_T_e_SG_D_3_eef6a) -> T_e_SG_D_3/1
  d_psi_1d_SG_D_3_block/1(Blockout_d_psi_1d_SG_D_3_db4c0) -> psi_1d_SG_D_3/1
  d_psi_gq_SG_D_3_block/1(Blockout_d_psi_gq_SG_D_3_d5302) -> psi_gq_SG_D_3/1
  d_psi_d_SG_D_3_block/1(Blockout_d_psi_d_SG_D_3_9ba56) -> psi_d_SG_D_3/1
  i_d_SG_D_3_block/1(Blockout_i_d_SG_D_3_fa4e4) -> i_d_SG_D_3/1
  i_q_SG_D_3_block/1(Blockout_i_q_SG_D_3_e7589) -> i_q_SG_D_3/1
  V_f_SG_D_3/1 -> d_V_f_SG_D_3_block/14(State_V_f_SG_D_3_0ee7b), d_E_fd_SG_D_3_block/2(State_V_f_SG_D_3_89c49)
  Px_3_SG_D_3/1 -> d_V_f_SG_D_3_block/3(State_Px_3_SG_D_3_c1107), d_Px_3_SG_D_3_block/1(State_Px_3_SG_D_3_af481)
  d_E_fd_SG_D_3_block/1(Blockout_d_E_fd_SG_D_3_cf470) -> E_fd_SG_D_3/1
  E_fd_SG_D_3/1 -> d_V_f_SG_D_3_block/1(State_E_fd_SG_D_3_d8376), d_E_fd_SG_D_3_block/1(State_E_fd_SG_D_3_7ac9b), d_psi_fd_SG_D_3_block/1(State_E_fd_SG_D_3_d78e2), d_R_f_SG_D_3_block/1(State_E_fd_SG_D_3_4b09f)
  d_psi_fd_SG_D_3_block/1(Blockout_d_psi_fd_SG_D_3_d4122) -> psi_fd_SG_D_3/1

== system IEEE14_case/SG_D_6 ==
  v_d_SG_D_6 : Inport
  v_q_SG_D_6 : Inport  Port=2
  E_fd_SG_D_6 : Integrator  InitialCondition=-0.10323140104081753
  Px_1_SG_D_6 : Integrator  InitialCondition=0.0
  Px_2_SG_D_6 : Integrator  InitialCondition=0.0
  Px_3_SG_D_6 : Integrator  InitialCondition=-7.053079060698743e-33
  R_f_SG_D_6 : Integrator  InitialCondition=-0.6969594304555766
  T_e_SG_D_6_block : Subsystem
  T_m_SG_D_6 : Integrator  InitialCondition=0.00041484947279289437
  V_f_SG_D_6 : Integrator  InitialCondition=-1.0323140104081752
  d_E_fd_SG_D_6_block : Subsystem
  d_Px_1_SG_D_6_block : Subsystem
  d_Px_2_SG_D_6_block : Subsystem
  d_Px_3_SG_D_6_block : Subsystem
  d_R_f_SG_D_6_block : Subsystem
  d_T_m_SG_D_6_block : Subsystem
  d_V_f_SG_D_6_block : Subsystem
  d_psi_1d_SG_D_6_block : Subsystem
  d_psi_d_SG_D_6_block : Subsystem
  d_psi_fd_SG_D_6_block : Subsystem
  d_psi_gq_SG_D_6_block : Subsystem
  d_psi_kq_SG_D_6_block : Subsystem
  d_psi_q_SG_D_6_block : Subsystem
  d_theta_SG_D_6_block : Subsystem
  d_w_SG_D_6_block : Subsystem
  i_d_SG_D_6_block : Subsystem
  i_q_SG_D_6_block : Subsystem
  psi_1d_SG_D_6 : Integrator  InitialCondition=1.0391238421429636
  psi_d_SG_D_6 : Integrator  InitialCondition=1.0699983081749576
  psi_fd_SG_D_6 : Integrator  InitialCondition=0.8835165333417134
  psi_gq_SG_D_6 : Integrator  InitialCondition=0.0012417752639932553
  psi_kq_SG_D_6 : Integrator  InitialCondition=-0.0019402738499894614
  psi_q_SG_D_6 : Integrator  InitialCondition=-0.0020178848039890396
  theta_SG_D_6 : Integrator  InitialCondition=-0.1647098511634469
  theta_SG_D_6_out_block : Subsystem
  w_SG_D_6 : Integrator  InitialCondition=376.99111843077515
  w_SG_D_6_out_block : Subsystem
  i_d_SG_D_6 : Outport
  i_q_SG_D_6 : Outport  Port=2
  T_e_SG_D_6 : Outport  Port=3
  w_SG_D_6_out : Outport  Port=4
  theta_SG_D_6_out : Outport  Port=5
  wires:
  w_SG_D_6/1 -> d_psi_d_SG_D_6_block/9(State_w_SG_D_6_f3bca), d_psi_q_SG_D_6_block/9(State_w_SG_D_6_19237), d_w_SG_D_6_block/1(State_w_SG_D_6_3de25), d_V_f_SG_D_6_block/8(State_w_SG_D_6_e114e), d_V_f_SG_D_6_block/13(State_w_SG_D_6_81790), d_Px_1_SG_D_6_block/2(State_w_SG_D_6_e1d55), d_theta_SG_D_6_block/1(State_w_SG_D_6_8d63a), d_Px_2_SG_D_6_block/4(State_w_SG_D_6_5d512), d_Px_3_SG_D_6_block/6(State_w_SG_D_6_5f02d), w_SG_D_6_out_block/1(State_w_SG_D_6_51261), d_T_m_SG_D_6_block/1(State_w_SG_D_6_e6164)
  d_Px_1_SG_D_6_block/1(Blockout_d_Px_1_SG_D_6_40901) -> Px_1_SG_D_6/1
  d_T_m_SG_D_6_block/1(Blockout_d_T_m_SG_D_6_83af8) -> T_m_SG_D_6/1
  w_SG_D_6_out_block/1(Blockout_w_SG_D_6_out_90215) -> w_SG_D_6_out/1
  T_m_SG_D_6/1 -> d_T_m_SG_D_6_block/2(State_T_m_SG_D_6_02315), d_w_SG_D_6_block/2(State_T_m_SG_D_6_5b3c9)
  d_Px_2_SG_D_6_block/1(Blockout_d_Px_2_SG_D_6_3663f) -> Px_2_SG_D_6/1
  d_w_SG_D_6_block/1(Blockout_d_w_SG_D_6_858c2) -> w_SG_D_6/1
  d_theta_SG_D_6_block/1(Blockout_d_theta_SG_D_6_40bf7) -> theta_SG_D_6/1
  i_q_SG_D_6_block/1(Blockout_i_q_SG_D_6_da8c6) -> i_q_SG_D_6/1
  d_Px_3_SG_D_6_block/1(Blockout_d_Px_3_SG_D_6_17e90) -> Px_3_SG_D_6/1
  d_psi_q_SG_D_6_block/1(Blockout_d_psi_q_SG_D_6_609ad) -> psi_q_SG_D_6/1
  psi_q_SG_D_6/1 -> d_psi_d_SG_D_6_block/8(State_psi_q_SG_D_6_65dc8), d_psi_q_SG_D_6_block/3(State_psi_q_SG_D_6_163e7), d_psi_gq_SG_D_6_block/6(State_psi_q_SG_D_6_acf1b), d_psi_gq_SG_D_6_block/9(State_psi_q_SG_D_6_63591), d_psi_kq_SG_D_6_block/5(State_psi_q_SG_D_6_e39b7), d_w_SG_D_6_block/6(State_psi_q_SG_D_6_bcef0), d_w_SG_D_6_block/7(State_psi_q_SG_D_6_5e3e6), d_V_f_SG_D_6_block/7(State_psi_q_SG_D_6_0a3e6), i_d_SG_D_6_block/3(State_psi_q_SG_D_6_db020), i_q_SG_D_6_block/3(State_psi_q_SG_D_6_d539d), T_e_SG_D_6_block/4(State_psi_q_SG_D_6_ac522), d_V_f_SG_D_6_block/11(State_psi_q_SG_D_6_83624), T_e_SG_D_6_block/5(State_psi_q_SG_D_6_09a29)
  psi_gq_SG_D_6/1 -> d_psi_q_SG_D_6_block/1(State_psi_gq_SG_D_6_ae354), d_psi_gq_SG_D_6_block/1(State_psi_gq_SG_D_6_9681f), d_psi_gq_SG_D_6_block/2(State_psi_gq_SG_D_6_f7256), d_psi_gq_SG_D_6_block/4(State_psi_gq_SG_D_6_8e9c1), d_psi_kq_SG_D_6_block/3(State_psi_gq_SG_D_6_38b04), d_w_SG_D_6_block/4(State_psi_gq_SG_D_6_45419), d_V_f_SG_D_6_block/9(State_psi_gq_SG_D_6_73017), d_psi_kq_SG_D_6_block/1(State_psi_gq_SG_D_6_1d13a), i_q_SG_D_6_block/1(State_psi_gq_SG_D_6_bb7cb), T_e_SG_D_6_block/2(State_psi_gq_SG_D_6_6e720), i_d_SG_D_6_block/1(State_psi_gq_SG_D_6_25250), d_psi_gq_SG_D_6_block/7(State_psi_gq_SG_D_6_45442)
  Px_2_SG_D_6/1 -> d_Px_2_SG_D_6_block/1(State_Px_2_SG_D_6_5cdcf), d_Px_3_SG_D_6_block/2(State_Px_2_SG_D_6_2857b), d_Px_3_SG_D_6_block/3(State_Px_2_SG_D_6_eb0dd)
  v_d_SG_D_6/1 -> d_psi_d_SG_D_6_block/4(Input_v_d_SG_D_6_af95d), d_psi_q_SG_D_6_block/4(Input_v_d_SG_D_6_c50dc)
  v_q_SG_D_6/1 -> d_psi_d_SG_D_6_block/6(Input_v_q_SG_D_6_c8c76), d_psi_q_SG_D_6_block/6(Input_v_q_SG_D_6_f6a8c)
  psi_fd_SG_D_6/1 -> d_psi_fd_SG_D_6_block/4(State_psi_fd_SG_D_6_4e3f4), d_psi_fd_SG_D_6_block/7(State_psi_fd_SG_D_6_38b04), d_psi_fd_SG_D_6_block/10(State_psi_fd_SG_D_6_10d72), d_V_f_SG_D_6_block/6(State_psi_fd_SG_D_6_fe54e), d_w_SG_D_6_block/10(State_psi_fd_SG_D_6_ba952), d_psi_fd_SG_D_6_block/2(State_psi_fd_SG_D_6_cff00), i_d_SG_D_6_block/7(State_psi_fd_SG_D_6_7efba), d_psi_1d_SG_D_6_block/5(State_psi_fd_SG_D_6_1aa59), d_psi_d_SG_D_6_block/3(State_psi_fd_SG_D_6_200cb), i_q_SG_D_6_block/7(State_psi_fd_SG_D_6_27308), d_psi_1d_SG_D_6_block/2(State_psi_fd_SG_D_6_9f319), T_e_SG_D_6_block/8(State_psi_fd_SG_D_6_b7b2b)
  psi_1d_SG_D_6/1 -> d_psi_fd_SG_D_6_block/8(State_psi_1d_SG_D_6_32df7), d_psi_d_SG_D_6_block/1(State_psi_1d_SG_D_6_101db), d_psi_fd_SG_D_6_block/5(State_psi_1d_SG_D_6_ebde4), d_psi_1d_SG_D_6_block/1(State_psi_1d_SG_D_6_c2ed2), d_psi_1d_SG_D_6_block/3(State_psi_1d_SG_D_6_eb113), d_psi_fd_SG_D_6_block/3(State_psi_1d_SG_D_6_bc672), d_w_SG_D_6_block/8(State_psi_1d_SG_D_6_cbb96), d_V_f_SG_D_6_block/4(State_psi_1d_SG_D_6_de2c8), i_q_SG_D_6_block/5(State_psi_1d_SG_D_6_399cf), T_e_SG_D_6_block/6(State_psi_1d_SG_D_6_60340), i_d_SG_D_6_block/5(State_psi_1d_SG_D_6_32fc9)
  d_psi_1d_SG_D_6_block/1(Blockout_d_psi_1d_SG_D_6_367d1) -> psi_1d_SG_D_6/1
  theta_SG_D_6/1 -> d_psi_d_SG_D_6_block/5(State_theta_SG_D_6_4b87e), d_psi_q_SG_D_6_block/5(State_theta_SG_D_6_a7791), i_d_SG_D_6_block/4(State_theta_SG_D_6_2ca6e), i_d_SG_D_6_block/8(State_theta_SG_D_6_5c117), i_q_SG_D_6_block/4(State_theta_SG_D_6_0f9f7), i_q_SG_D_6_block/8(State_theta_SG_D_6_711a7), theta_SG_D_6_out_block/1(State_theta_SG_D_6_29a7d), d_psi_q_SG_D_6_block/7(State_theta_SG_D_6_9e13e), d_psi_d_SG_D_6_block/7(State_theta_SG_D_6_acea8)
  d_E_fd_SG_D_6_block/1(Blockout_d_E_fd_SG_D_6_64fbc) -> E_fd_SG_D_6/1
  psi_kq_SG_D_6/1 -> d_psi_q_SG_D_6_block/2(State_psi_kq_SG_D_6_fbd08), d_psi_gq_SG_D_6_block/3(State_psi_kq_SG_D_6_591fc), d_psi_gq_SG_D_6_block/5(State_psi_kq_SG_D_6_f7f8f), d_psi_gq_SG_D_6_block/8(State_psi_kq_SG_D_6_32c36), d_psi_kq_SG_D_6_block/4(State_psi_kq_SG_D_6_0165b), d_V_f_SG_D_6_block/10(State_psi_kq_SG_D_6_ef584), i_d_SG_D_6_block/2(State_psi_kq_SG_D_6_05164), i_q_SG_D_6_block/2(State_psi_kq_SG_D_6_74fba), d_psi_kq_SG_D_6_block/2(State_psi_kq_SG_D_6_a092f), T_e_SG_D_6_block/3(State_psi_kq_SG_D_6_3291f), d_w_SG_D_6_block/5(State_psi_kq_SG_D_6_9cfe6)
  Px_1_SG_D_6/1 -> d_Px_2_SG_D_6_block/3(State_Px_1_SG_D_6_357af), d_Px_1_SG_D_6_block/1(State_Px_1_SG_D_6_18725), d_Px_3_SG_D_6_block/4(State_Px_1_SG_D_6_c3a44), d_Px_3_SG_D_6_block/5(State_Px_1_SG_D_6_b27f4), d_Px_2_SG_D_6_block/2(State_Px_1_SG_D_6_26ff3)
  d_V_f_SG_D_6_block/1(Blockout_d_V_f_SG_D_6_09efe) -> V_f_SG_D_6/1
  psi_d_SG_D_6/1 -> d_psi_fd_SG_D_6_block/6(State_psi_d_SG_D_6_92222), d_psi_fd_SG_D_6_block/9(State_psi_d_SG_D_6_beaed), d_psi_q_SG_D_6_block/8(State_psi_d_SG_D_6_700ce), d_w_SG_D_6_block/3(State_psi_d_SG_D_6_61dab), i_d_SG_D_6_block/6(State_psi_d_SG_D_6_8fce8), d_V_f_SG_D_6_block/12(State_psi_d_SG_D_6_91b9a), d_psi_1d_SG_D_6_block/4(State_psi_d_SG_D_6_4a5c3), d_V_f_SG_D_6_block/5(State_psi_d_SG_D_6_cf70a), i_q_SG_D_6_block/6(State_psi_d_SG_D_6_c39a1), d_psi_d_SG_D_6_block/2(State_psi_d_SG_D_6_c802b), d_w_SG_D_6_block/9(State_psi_d_SG_D_6_2f7e7), T_e_SG_D_6_block/1(State_psi_d_SG_D_6_50e5d), T_e_SG_D_6_block/7(State_psi_d_SG_D_6_bc7a5)
  T_e_SG_D_6_block/1(Blockout_T_e_SG_D_6_1c5ce) -> T_e_SG_D_6/1
  R_f_SG_D_6/1 -> d_V_f_SG_D_6_block/2(State_R_f_SG_D_6_28e1c), d_R_f_SG_D_6_block/2(State_R_f_SG_D_6_39afc)
  d_psi_gq_SG_D_6_block/1(Blockout_d_psi_gq_SG_D_6_58558) -> psi_gq_SG_D_6/1
  d_psi_d_SG_D_6_block/1(Blockout_d_psi_d_SG_D_6_3b081) -> psi_d_SG_D_6/1
  d_R_f_SG_D_6_block/1(Blockout_d_R_f_SG_D_6_b769e) -> R_f_SG_D_6/1
  d_psi_kq_SG_D_6_block/1(Blockout_d_psi_kq_SG_D_6_f15a3) -> psi_kq_SG_D_6/1
  Px_3_SG_D_6/1 -> d_Px_3_SG_D_6_block/1(State_Px_3_SG_D_6_9df2d), d_V_f_SG_D_6_block/3(State_Px_3_SG_D_6_bef29)
  theta_SG_D_6_out_block/1(Blockout_theta_SG_D_6_out_e355f) -> theta_SG_D_6_out/1
  i_d_SG_D_6_block/1(Blockout_i_d_SG_D_6_c0693) -> i_d_SG_D_6/1
  V_f_SG_D_6/1 -> d_V_f_SG_D_6_block/14(State_V_f_SG_D_6_82040), d_E_fd_SG_D_6_block/2(State_V_f_SG_D_6_97849)
  E_fd_SG_D_6/1 -> d_R_f_SG_D_6_block/1(State_E_fd_SG_D_6_ceac9), d_V_f_SG_D_6_block/1(State_E_fd_SG_D_6_02805), d_psi_fd_SG_D_6_block/1(State_E_fd_SG_D_6_8c2c7), d_E_fd_SG_D_6_block/1(State_E_fd_SG_D_6_93beb)
  d_psi_fd_SG_D_6_block/1(Blockout_d_psi_fd_SG_D_6_50674) -> psi_fd_SG_D_6/1
